simulink model "DFIGStatorVoltageDrop"  (R2013a)
settings: Solver=ode45  StartTime=0.0  StopTime=10.0  RelTol=1e-3
libraries: powerlib x5, re_lib x1
settings Model: Creator=Sony  LastModifiedBy=Sony

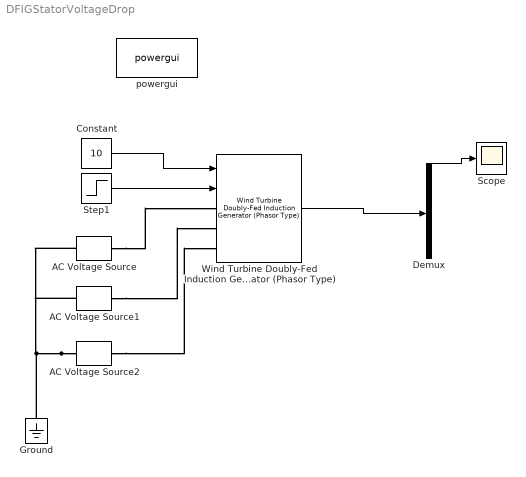
== system DFIGStatorVoltageDrop ==
  AC Voltage Source : powerlib/Electrical Sources/AC Voltage Source  Amplitude=563.38264  Phase=90  Frequency=50  SampleTime=0  Measurements=None
  AC Voltage Source1 : powerlib/Electrical Sources/AC Voltage Source  Amplitude=563.38264  Phase=-30  Frequency=50  SampleTime=0  Measurements=None
  AC Voltage Source2 : powerlib/Electrical Sources/AC Voltage Source  Amplitude=563.38264  Phase=-150  Frequency=50  SampleTime=0  Measurements=None
  Constant : Constant  Value=10
  Demux : Demux  Outputs=20
  Ground : powerlib/Elements/Ground  LConnTagsString=a
  Scope : Scope
  Step1 : Step  Time=0  SampleTime=0
  Wind Turbine Doubly-Fed Induction Generator (Phasor Type) : re_lib/Wind Generation/Wind Turbine Doubly-Fed Induction Generator (Phasor Type)  ShowParameters=Generator data  nom=[1.5e6/0.9 575 60]  sta=[ 0.00706 0.171]  rot=[ 0.005 0.156]  Lm=2.9  mec=[5.04 0.01 3]  init=[0.2 0 0 0 0 0]  Pmax=0.5  Lchoke=[0.15 0.15/100]  init_inductor=[0 90]  Vdc_nom=1200  capacitor=10000e-6  ExternalTm=off  DisplayTurbChar=off  speed_power=[0 0; 0.24 0.007; 0.36 0.024; 0.6 0.112; 0.96 0.46; 1.2 0.898; 1.5 0.898]  Pmec=1.5e6  speed_ABCD=[0.7 0.71 1.2 1.21]  power_C=0.73  wind_point_C=12  pitch_gain=500  pitch_max=45  pitch_rate=2  ControlVQ=Voltage regulation  ExternalVref=off  Vref=1.0  ExternalQref=off  Qref=0  ExternalIqref=off  Iq_ref=0  Kpi_volt_reg=[1.25 300]  Xs=0.02  Kpi_Q=[0.05 5]  Kpi_power_reg=[1 100]  Kpi_dc_reg=[0.002 0.05]  Kpi_grid_side_cur_reg=[1 100]  Kpi_rotor_side_cur_reg=[0.3 8]  V_slew_rate=100  Q_slew_rate=100  power_slew_rate=1  current_slew_rate=200
  powergui : powerlib/powergui  Priority=1  SimulationMode=Phasor  SolverType=Tustin  SampleTime=50e-6  frequency=50  SPID=off  DisableSnubberDevices=off  DisableRonSwitches=off  DisableVfSwitches=off  SwTol=0  Interpol=off  DisplayEquations=off  frequencyindice=50  Pbase=100e6  ErrMax=1e-4  Iterations=50  UnitsV=kV  UnitsW=MW  FunctionMessages=off  echomessages=off  HookPort=off  EnableUseOfTLC=off  x0status=blocks  RestoreLinks=warning  ResistiveCurrentMeasurement=off  Frange=[0:2:500]  Ylog=off  Xlog=on  ShowGrid=off  save=off  variable=ZData  ZoomFFT=off  StartTime=0.0  cycles=1  DisplayStyle=1  fundamental=60  FreqAxis=off  MaxFrequency=1000  frequencyindicesteady=1  RmsSteady=1  display=off  Ts=0  methode=off
  wires:
  Step1/1 -> Wind Turbine Doubly-Fed Induction Generator (Phasor Type)/2
  Constant/1 -> Wind Turbine Doubly-Fed Induction Generator (Phasor Type)/1
  Wind Turbine Doubly-Fed Induction Generator (Phasor Type)/1 -> Demux/1
  Demux/1 -> Scope/1
  connections:
  AC Voltage Source2/LConn1 -- AC Voltage Source/LConn1 -- AC Voltage Source1/LConn1 -- Ground/LConn1
  AC Voltage Source/RConn1 -- Wind Turbine Doubly-Fed Induction Generator (Phasor Type)/LConn1
  AC Voltage Source1/RConn1 -- Wind Turbine Doubly-Fed Induction Generator (Phasor Type)/LConn2
  AC Voltage Source2/RConn1 -- Wind Turbine Doubly-Fed Induction Generator (Phasor Type)/LConn3
